simulink model "t_validation_V2_19b"  (R2019b)
settings: Solver=VariableStepAuto  StartTime=0.0  StopTime=200  RelTol=1e-3
model workspace (MAT data in the model file):
  x2xx = 0
values from neighbouring files (symbols this model uses):
  KDspd = 0    [time_validation.m]
  KIspd = 0    [time_validation.m]
  KPspd = 20    [time_validation.m]
  Q0 = zeros(Nu+2,1)    [time_validation.m]
  QD0 = Q0    [time_validation.m]
  v_ref = vconst    (= 5.55555555556)    [time_validation.m]
undefined symbols (not defined in the file or in its folder): axle_rate_limit, Lspd, Nspd, PARSa, PARSu, Tmc, Uspd
libraries: simulink x2
(part 3 of 3)

== matlab function t_validation_V2_19b/time-domain-test/double-general-nonlineartyre-nonlinear-variable-matrix/Tau_tire ==
  data: q input; qd input; delta input; Fx input; Tau_tire output; Alpha output
function [Tau_tire, Alpha] = calculate_Tau_tire(q, qd, delta, Fx)

% coefficient

l_j1j2 = 11.4;
l_j2j3 = 9.4;
l_j1a1 = 2.5;
l_j1a2 = 4;
l_j1a3 = 9.9;
l_j2a4 = 1.5;
l_j2a5 = 7.9;
l_j3a6 = 1.5;
l_j3a7 = 7.4;
l_j3a8 = 8.9;
h11 = 0.9625;
h12 = 0.9625;
h13 = 0.98;
h21 = 0.98; 
h22 = 0.98;
h31 = 0.98;
h32 = 0.9625;
h33 = 0.9625;

x = q(1);
y = q(2);
psi1 = q(3);
psi2 = q(4);
psi3 = q(5);
xd = qd(1);
yd = qd(2);
psi1d = qd(3);
psi2d = qd(4);
psi3d = qd(5);

psij = [psi1, psi2, psi3]';
Rot_w2v = zeros(2, 2, 3);
for i = 1:3
    Rot_w2v(:, :, i) = [cos(psij(i)), -sin(psij(i));
                        sin(psij(i)), cos(psij(i));];
end

Rot_v2t = zeros(2, 2, 8);
for i = 1:8
    Rot_v2t(:, :, i) = [cos(delta(i)), -sin(delta(i));
                        sin(delta(i)), cos(delta(i));];
end

xj = zeros(3, 1);
yj = zeros(3, 1);
xj(1) = x;
yj(1) = y;
xj(2) = x - l_j1j2*cos(psi1);
yj(2) = y - l_j1j2*sin(psi1);
xj(3) = x - l_j1j2*cos(psi1) - l_j2j3*cos(psi2);
yj(3) = y - l_j1j2*sin(psi1) - l_j2j3*sin(psi2);

u = zeros(2, 3);
n = zeros(2, 3);
for i = 1:3
    u(:, i)=[cos(q(i + 2)), sin(q(i + 2))]';
    n(:, i)=[-sin(q(i + 2)), cos(q(i + 2))]';
end

IU = [1, 1, 1, 2, 2, 3, 3, 3]';
l_ja = [l_j1a1, l_j1a2, l_j1a3, l_j2a4, l_j2a5, l_j3a6, l_j3a7, l_j3a8]';
ha = [h11, h12, h13, h21, h22, h31, h32, h33]';

L_long1 = [cos(psi1), cos(psi1), cos(psi1), cos(psi2), cos(psi2), cos(psi3), cos(psi3), cos(psi3);
           sin(psi1), sin(psi1), sin(psi1), sin(psi2), sin(psi2), sin(psi3), sin(psi3), sin(psi3);
           -h11, -h12, -h13, l_j1j2*sin(psi1-psi2), l_j1j2*sin(psi1-psi2), l_j1j2*sin(psi1-psi3), l_j1j2*sin(psi1-psi3), l_j1j2*sin(psi1-psi3);
           0, 0, 0, -h21, -h22, l_j2j3*sin(psi2-psi3), l_j2j3*sin(psi2-psi3), l_j2j3*sin(psi2-psi3);
           0, 0, 0, 0, 0, -h31, -h32, -h33;];

L_long2 = [cos(psi1), cos(psi1), cos(psi1), cos(psi2), cos(psi2), cos(psi3), cos(psi3), cos(psi3);
           sin(psi1), sin(psi1), sin(psi1), sin(psi2), sin(psi2), sin(psi3), sin(psi3), sin(psi3);
           h11, h12, h13, l_j1j2*sin(psi1-psi2), l_j1j2*sin(psi1-psi2), l_j1j2*sin(psi1-psi3), l_j1j2*sin(psi1-psi3), l_j1j2*sin(psi1-psi3);
           0, 0, 0, h21, h22, l_j2j3*sin(psi2-psi3), l_j2j3*sin(psi2-psi3), l_j2j3*sin(psi2-psi3);
           0, 0, 0, 0, 0, h31, h32, h33;];

L_lat1 = [-sin(psi1), -sin(psi1), -sin(psi1), -sin(psi2), -sin(psi2), -sin(psi3), -sin(psi3), -sin(psi3);
          cos(psi1), cos(psi1), cos(psi1), cos(psi2), cos(psi2), cos(psi3), cos(psi3), cos(psi3);
          -l_j1a1, -l_j1a2, -l_j1a3, -l_j1j2*cos(psi1-psi2), -l_j1j2*cos(psi1-psi2), -l_j1j2*cos(psi1-psi3), -l_j1j2*cos(psi1-psi3), -l_j1j2*cos(psi1-psi3);
          0, 0, 0, -l_j2a4, -l_j2a5, -l_j2j3*cos(psi2-psi3), -l_j2j3*cos(psi2-psi3), -l_j2j3*cos(psi2-psi3);
          0, 0, 0, 0, 0, -l_j3a6, -l_j3a7, -l_j3a8;];

L_lat2 = [-sin(psi1), -sin(psi1), -sin(psi1), -sin(psi2), -sin(psi2), -sin(psi3), -sin(psi3), -sin(psi3);
          cos(psi1), cos(psi1), cos(psi1), cos(psi2), cos(psi2), cos(psi3), cos(psi3), cos(psi3);
          -l_j1a1, -l_j1a2, -l_j1a3, -l_j1j2*cos(psi1-psi2), -l_j1j2*cos(psi1-psi2), -l_j1j2*cos(psi1-psi3), -l_j1j2*cos(psi1-psi3), -l_j1j2*cos(psi1-psi3);
          0, 0, 0, -l_j2a4, -l_j2a5, -l_j2j3*cos(psi2-psi3), -l_j2j3*cos(psi2-psi3), -l_j2j3*cos(psi2-psi3);
          0, 0, 0, 0, 0, -l_j3a6, -l_j3a7, -l_j3a8;];

Delta_c = zeros(8, 8);
Delta_s = zeros(8, 8);
for i = 1:8
    Delta_c(i, i) = cos(delta(i));
    Delta_s(i, i) = sin(delta(i));
end

vxj = zeros(3, 1);
vyj = zeros(3, 1);
vxj(1) = xd;
vyj(1) = yd;
vxj(2) = xd + l_j1j2*sin(psi1)*psi1d;
vyj(2) = yd - l_j1j2*cos(psi1)*psi1d;
vxj(3) = xd + l_j1j2*sin(psi1)*psi1d + l_j2j3*sin(psi2)*psi2d;
vyj(3) = yd - l_j1j2*cos(psi1)*psi1d - l_j2j3*cos(psi2)*psi2d;
va1 = zeros(2, 8);
va2 = zeros(2, 8);
psidj = [psi1d, psi2d, psi3d]';
for i = 1:8
    va1(:, i) = [vxj(IU(i)); vyj(IU(i))] - n(:, IU(i))*l_ja(i)*psidj(IU(i)) + (-1)*u(:, IU(i))*ha(i)*psidj(IU(i));
    va2(:, i) = [vxj(IU(i)); vyj(IU(i))] - n(:, IU(i))*l_ja(i)*psidj(IU(i)) + u(:, IU(i))*ha(i)*psidj(IU(i));
end

va1_v = zeros(2, 8);
va2_v = zeros(2, 8);
for i = 1:8
    va1_v(:, i) = inv(Rot_w2v(:, :, IU(i)))*va1(:, i);
    va2_v(:, i) = inv(Rot_w2v(:, :, IU(i)))*va2(:, i);
end

beta1 = zeros(8, 1);
beta2 = zeros(8, 1);
for i = 1:8
    beta1(i) = atan2(va1_v(2, i), va1_v(1, i));
    beta2(i) = atan2(va2_v(2, i), va2_v(1, i));
end

% magic formula
% 魔术公式参数
A = [1.65, -34, 1250, 4535, 12.8, 0.00501, -0.02103,  0.77394, ...
     0.0022890, 0.013442, 0.003709, 19.1656, 1.21356, 6.26206]';

% 轮胎垂向载荷 kN
Fz = 30000 / 1000;

Fy1 = zeros(8, 1);
Fy2 = zeros(8, 1);
gamma = 0;
for i = 1:8
    alpha = (delta(i) - beta1(i)) * 180 / pi;
    Sh = A(10) * Fz + A(11) + A(9) * gamma;
    Sv = A(12) * Fz * gamma + A(13) * Fz + A(14);
    C = A(1);
    D = A(2) * Fz ^ 2 + A(3) * Fz;
    BCD = A(4) * sin(2 * atan(Fz / A(5))) * (1 - A(6) * abs(gamma));
    B = BCD / (C * D);
    E = A(7) * Fz + A(8);
    x = alpha; % + Sh;
    % 轮胎侧向力
    Fy1(i) = D * sin(C * atan(B * x - E * (B * x - atan(B * x)))); % + Sv;
end
for i = 1:8
    alpha = (delta(i) - beta2(i)) * 180 / pi;
    Sh = A(10) * Fz + A(11) + A(9) * gamma;
    Sv = A(12) * Fz * gamma + A(13) * Fz + A(14);
    C = A(1);
    D = A(2) * Fz ^ 2 + A(3) * Fz;
    BCD = A(4) * sin(2 * atan(Fz / A(5))) * (1 - A(6) * abs(gamma));
    B = BCD / (C * D);
    E = A(7) * Fz + A(8);
    x = alpha; % + Sh;
    % 轮胎侧向力
    Fy2(i) = D * sin(C * atan(B * x - E * (B * x - atan(B * x)))); % + Sv;
end

Tau_tire = L_long1 * (Delta_c * Fx / 2 - Delta_s * Fy1) ...
         + L_long2 * (Delta_c * Fx / 2 - Delta_s * Fy2) ...
         + L_lat1 * (Delta_s * Fx / 2 + Delta_c * Fy1) ...
         + L_lat2 * (Delta_s * Fx / 2 + Delta_c * Fy2);

beta = (beta1 + beta2) / 2;
Alpha = delta - beta;

end

== matlab function t_validation_V2_19b/time-domain-test/double-general-nonlineartyre-nonlinear-variable-matrix/qdd ==
  data: M input; C input; D input; qd input; Q input; qdd output
function qdd = calculate_qdd(M, C, D, qd, Q)

qdd = inv(M)*(Q - C * qd - D * qd);

end

== matlab function t_validation_V2_19b/time-domain-test/ Motion Controller2/discrete-time subsystem/MATLAB Function ==
  data: str1 input; y output; PARSa input
function y = StrMux(str1,PARSa)
%distribute steering from driver (and auto steer in future versions)
y=PARSa(:,6);
y=y*str1;
end

== matlab function t_validation_V2_19b/time-domain-test/ Motion Controller2/discrete-time subsystem/MATLAB Function1 ==
  data: adem input; y output; PARSu input; PARSa input
function y = wheel_force_distibution(adem,PARSu,PARSa)

y=zeros(8,1); 
mass=sum(PARSu(:,1));
Na=size(PARSa,1);
if adem>0
    y(1:Na)=PARSa(:,4); %drive axle distribution
else
    y(1:Na)=PARSa(:,5); %brake force distribution
end
n=sum(y);
y=y*mass*adem/n;
end

== matlab function t_validation_V2_19b/time-domain-test/ Motion Controller1/discrete-time subsystem/MATLAB Function ==
  data: str1 input; y output; PARSa input
function y = StrMux(str1,PARSa)
%distribute steering from driver (and auto steer in future versions)
y=PARSa(:,6);
y=y*str1;
end

== matlab function t_validation_V2_19b/time-domain-test/ Motion Controller2/discrete-time subsystem/find_vx1 ==
  settings: updateMethod=DISCRETE
  data: vx6 output; q input; qd input
function vx6 = vx_conversion(q,qd)
%#codegen
% convert q and qd to vx6 needed for the driver model

xxp=2; %nominal point P of driver 
u1=[cos(q(3));sin(q(3))];n1=[-sin(q(3));cos(q(3))];
rp = q(1:2)-xxp*u1;

v00=qd(1:2); %global velocity at front joint
vp=v00-qd(3)*xxp*n1; %move to driver point
U=dot(vp,u1);V=dot(vp,n1); %components in body axes (unit 1)
vx6=[U;V;qd(3);rp;q(3)]; %standard format ... [U,V,r,x,y,psi]'
end

== matlab function t_validation_V2_19b/time-domain-test/double-general-lineartyre-nonlinear-variable-matrix1/状态输入 ==
  data: steer input; sign output; fx input
function sign = is_start(steer, fx)

sign = 1;
if steer == zeros(8,1) 
    if fx == zeros(8,1)
        sign = 0;
    end
end

end
